simulink model "sampleModel1510_1_sub_sub"  (R2023a)
settings: Solver=VariableStepAuto  StartTime=0.0  StopTime=10.0  RelTol=1e-3
libraries: simulink x3, hdlsllib x1
settings Model: Creator=user1  LastModifiedBy=user1
settings OptimizationCC: BlockReduction=off  ConditionallyExecuteInputs=off

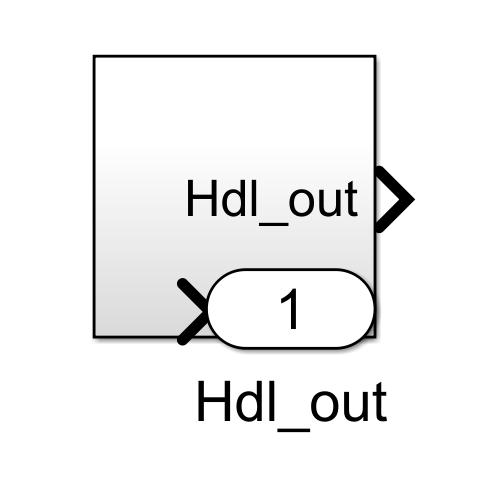
[thumbnail: Simulink's stored preview of the top-level diagram]
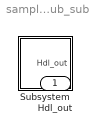
== system sampleModel1510_1_sub_sub ==
  Subsystem : Subsystem
  Hdl_out : Outport  OutDataTypeStr=uint8

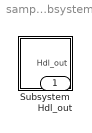
== system sampleModel1510_1_sub_sub/Subsystem ==
  Subsystem : Subsystem
  Hdl_out : Outport  OutDataTypeStr=uint8

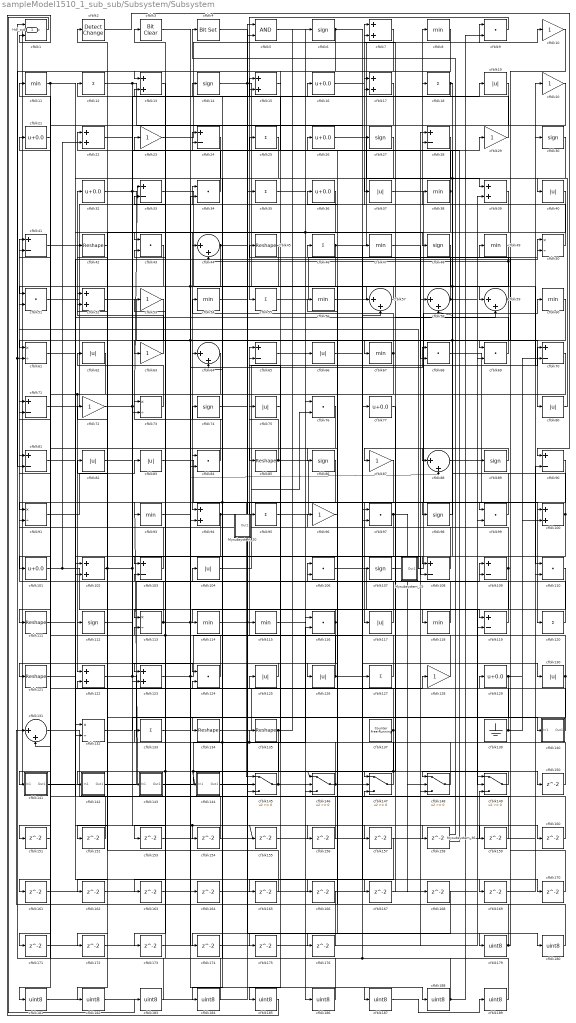
== system sampleModel1510_1_sub_sub/Subsystem/Subsystem ==
  Mysubsystem_20 : Subsystem  TreatAsAtomicUnit=on  RTWFcnName=Mysubsystem_20
      settings: RTWFcnNameOpts=User specified  RTWFileNameOpts=Use function name
  Mysubsystem_25 : Subsystem  TreatAsAtomicUnit=on  RTWFcnName=Mysubsystem_25
      settings: RTWFcnNameOpts=User specified  RTWFileNameOpts=Use function name
  Mysubsystem_36 : Subsystem  TreatAsAtomicUnit=on  RTWFcnName=Mysubsystem_36
      settings: RTWFcnNameOpts=User specified  RTWFileNameOpts=Use function name
  cfblk1 : RelationalOperator  Operator=<=  OutDataTypeStr=boolean  InputSameDT=off
  cfblk{10,20,23,29,53,63,72,87,96,128} (10 alike) : Gain  OutDataTypeStr=uint8
  cfblk{7,13,15,17,22,39,52,94,100,102,122..123} (12 alike) : Sum  OutDataTypeStr=uint8
  cfblk{16,21,26,32,36,77,101,129} (8 alike) : Bias  Bias=0.0  SaturateOnIntegerOverflow=off
  cfblk{24,28,33,41,65,70..71,81,90,103,108..109,119} (13 alike) : Sum  Inputs=+-  OutDataTypeStr=uint8
  cfblk{19,37,40,62,66,75,80,82..83,104,117,125..126,130} (14 alike) : Abs  OutDataTypeStr=uint8  SaturateOnIntegerOverflow=off
  cfblk{9,34,43,51,68..69,76,84,97,99,106,110,116,124} (14 alike) : DotProduct  OutDataTypeStr=uint8
  cfblk{6,14,27,30,48,74,86,89,98,107,112} (11 alike) : Signum
  cfblk{8,11,38,47,49,54,56,60,67,93,114..115,118} (13 alike) : MinMax  OutDataTypeStr=uint8
  cfblk{42,45,85,111,121,134..135} (7 alike) : Reshape
  cfblk{50,61,73,91,113,132} (6 alike) : Product  Inputs=*/  OutDataTypeStr=uint8  RndMeth=Zero  SaturateOnIntegerOverflow=on
  cfblk{12,18,25,35,46,55,95,120,127,133} (10 alike) : Sum  Inputs=+  OutDataTypeStr=uint8
  cfblk{44,57..59,64,88,131} (7 alike) : Sum  Inputs=|++  OutDataTypeStr=uint8
  cfblk137 : hdlsllib/Sources/Counter Free-Running  NumBits=16  tsamp=-1
  cfblk139 : Ground
  cfblk140 : Subsystem
      settings: LibrarySourceBlock=|
      | hdlsllib/Ports &
      | Subsystems/Subsystem
  cfblk141 : Subsystem
      settings: LibrarySourceBlock=|
      | hdlsllib/Ports &
      | Subsystems/Subsystem
  cfblk142 : Subsystem
      settings: LibrarySourceBlock=|
      | hdlsllib/Ports &
      | Subsystems/Subsystem
  cfblk143 : Subsystem
      settings: LibrarySourceBlock=|
      | hdlsllib/Ports &
      | Subsystems/Subsystem
  cfblk144 : Subsystem
      settings: LibrarySourceBlock=|
      | hdlsllib/Ports &
      | Subsystems/Subsystem
  cfblk{145..149} (5 alike) : Switch  OutDataTypeStr=uint8  SaturateOnIntegerOverflow=off  InputSameDT=off
  cfblk{150..176} (27 alike) : Delay  SampleTime=1
  cfblk{179..189} (11 alike) : DataTypeConversion  OutDataTypeStr=uint8  SaturateOnIntegerOverflow=off  RndMeth=Floor
  cfblk2 : simulink/Logic and Bit Operations/Detect Change  vinit=0  OutDataTypeStr=uint8
      settings: LibrarySourceBlock=|
      | hdlsllib/Logic and Bit
      | Operations/Detect
      | Change
  cfblk3 : simulink/Logic and Bit Operations/Bit Clear  iBit=0
      settings: LibrarySourceBlock=|
      | hdlsllib/Logic and Bit
      | Operations/Bit Clear
  cfblk4 : simulink/Logic and Bit Operations/Bit Set  iBit=0
      settings: LibrarySourceBlock=|
      | hdlsllib/Logic and Bit
      | Operations/Bit Set
  cfblk5 : Logic  AllPortsSameDT=off  OutDataTypeStr=boolean
  Hdl_out : Outport  OutDataTypeStr=uint8
  wires:
  Mysubsystem_36/2(Out2) -> cfblk23/1
  Mysubsystem_36/1(Out1) -> cfblk4/1
  Mysubsystem_25/1(Out1) -> cfblk51/2
  Mysubsystem_20/1(Out1) -> cfblk76/2
  cfblk189/1 -> cfblk133/1
  cfblk187/1 -> cfblk189/1
  cfblk188/1 -> cfblk97/1, cfblk74/1, cfblk9/2
  cfblk3/1 -> cfblk187/1
  cfblk186/1 -> cfblk3/1
  cfblk65/1 -> cfblk186/1
  cfblk185/1 -> cfblk1/2
  cfblk157/1 -> cfblk185/1
  cfblk184/1 -> cfblk1/1
  cfblk168/1 -> cfblk184/1
  cfblk183/1 -> cfblk21/1
  cfblk1/1 -> cfblk183/1
  cfblk182/1 -> cfblk5/2
  cfblk42/1 -> cfblk182/1
  cfblk181/1 -> cfblk5/1
  cfblk87/1 -> cfblk181/1
  cfblk180/1 -> cfblk36/1
  cfblk5/1 -> cfblk180/1
  cfblk179/1 -> cfblk113/2, cfblk129/1
  cfblk176/1 -> cfblk64/2
  cfblk175/1 -> cfblk58/1
  cfblk75/1 -> cfblk175/1
  cfblk174/1 -> cfblk148/3
  cfblk173/1 -> cfblk57/2
  cfblk172/1 -> cfblk39/2
  cfblk70/1 -> cfblk172/1
  cfblk171/1 -> cfblk34/2
  cfblk170/1 -> cfblk109/2
  cfblk169/1 -> cfblk110/2
  cfblk167/1 -> cfblk147/3
  cfblk166/1 -> cfblk131/1
  cfblk61/1 -> cfblk166/1
  cfblk165/1 -> cfblk122/2
  cfblk164/1 -> cfblk99/2
  cfblk93/1 -> cfblk164/1
  cfblk163/1 -> cfblk69/2
  cfblk162/1 -> cfblk149/1
  cfblk36/1 -> cfblk162/1
  cfblk161/1 -> cfblk28/1
  cfblk43/1 -> cfblk161/1
  cfblk160/1 -> cfblk7/2
  cfblk115/1 -> cfblk160/1
  cfblk159/1 -> cfblk71/2
  cfblk158/1 -> cfblk149/3
  cfblk156/1 -> cfblk132/1
  cfblk112/1 -> cfblk156/1
  cfblk155/1 -> cfblk97/2
  cfblk154/1 -> cfblk41/2
  cfblk153/1 -> cfblk90/2
  cfblk152/1 -> cfblk102/1
  cfblk151/1 -> cfblk91/2
  cfblk20/1 -> cfblk151/1
  cfblk150/1 -> cfblk65/2
  cfblk74/1 -> cfblk150/1
  cfblk137/1 -> cfblk73/1, cfblk146/3
  cfblk19/1 -> cfblk147/2
  cfblk64/1 -> cfblk131/2
  cfblk48/1 -> cfblk101/1
  cfblk97/1 -> cfblk102/2, cfblk148/2
  cfblk108/1 -> cfblk42/1
  cfblk148/1 -> cfblk135/1, cfblk82/1
  cfblk118/1 -> cfblk52/1
  cfblk119/1 -> cfblk13/2
  cfblk4/1 -> cfblk179/1
  cfblk28/1 -> cfblk37/1
  cfblk69/1 -> cfblk27/1
  cfblk60/1 -> cfblk113/1, cfblk84/2, cfblk108/1
  cfblk22/1 -> cfblk19/1
  cfblk88/1 -> cfblk89/1
  cfblk121/1 -> cfblk59/2
  cfblk2/1 -> cfblk90/1
  cfblk96/1 -> cfblk56/1
  cfblk7/1 -> cfblk85/1
  cfblk82/1 -> cfblk34/1
  cfblk47/1 -> cfblk68/2
  cfblk130/1 -> cfblk106/2, cfblk145/3
  cfblk49/1 -> cfblk58/2, cfblk176/1
  cfblk114/1 -> cfblk18/1, cfblk158/1
  cfblk29/1 -> cfblk2/1
  cfblk111/1 -> cfblk50/1
  cfblk126/1 -> cfblk53/1, cfblk11/1, cfblk169/1
  cfblk11/1 -> cfblk111/1, cfblk44/1
  cfblk40/1 -> cfblk145/2
  cfblk124/1 -> cfblk33/2
  cfblk30/1 -> cfblk84/1, cfblk88/1
  cfblk134/1 -> cfblk57/1
  cfblk135/1 -> cfblk152/1, cfblk153/1, cfblk6/1
  cfblk120/1 -> cfblk104/1
  cfblk103/1 -> cfblk81/1
  cfblk33/1 -> cfblk76/1
  cfblk66/1 -> cfblk130/1
  cfblk41/1 -> cfblk48/1
  cfblk67/1 -> cfblk54/1, cfblk163/1
  cfblk98/1 -> cfblk28/2
  cfblk76/1 -> cfblk141/1(In1)
  cfblk52/1 -> cfblk80/1
  cfblk34/1 -> cfblk12/1
  cfblk55/1 -> cfblk20/1
  cfblk8/1 -> cfblk61/2, cfblk81/2
  cfblk59/1 -> cfblk45/1, cfblk44/2, cfblk86/1
  cfblk100/1 -> cfblk24/1, cfblk123/1
  cfblk84/1 -> cfblk43/2
  cfblk57/1 -> cfblk51/1
  cfblk123/1 -> cfblk47/1, cfblk88/2
  cfblk26/1 -> cfblk39/1
  cfblk143/1(Out1) -> cfblk116/2, cfblk35/1, cfblk146/1
  cfblk109/1 -> cfblk14/1, cfblk165/1
  cfblk132/1 -> cfblk140/1(In1)
  cfblk80/1 -> cfblk40/1
  cfblk113/1 -> cfblk68/1, cfblk167/1, cfblk52/2
  cfblk91/1 -> cfblk83/1
  cfblk53/1 -> cfblk61/1
  cfblk85/1 -> cfblk127/1, cfblk75/1
  cfblk38/1 -> cfblk64/1, cfblk15/1
  cfblk99/1 -> cfblk25/1
  cfblk102/1 -> cfblk29/1, cfblk119/1, cfblk72/1
  cfblk23/1 -> cfblk9/1
  cfblk12/1 -> cfblk77/1, cfblk108/2
  cfblk101/1 -> cfblk149/2, cfblk22/2
  cfblk32/1 -> cfblk66/1, cfblk124/1
  cfblk25/1 -> cfblk134/1
  cfblk149/1 -> cfblk148/1
  cfblk146/1 -> cfblk62/1, cfblk124/2, cfblk70/1
  cfblk144/1(Out1) -> cfblk17/2
  cfblk44/1 -> cfblk94/2, cfblk123/2, cfblk107/1
  cfblk17/1 -> cfblk43/1
  cfblk110/1 -> cfblk126/1
  cfblk10/1 -> cfblk69/1
  cfblk145/1 -> cfblk103/2, cfblk159/1, Hdl_out/1
  cfblk21/1 -> cfblk91/1
  cfblk141/1(Out1) -> cfblk128/1
  cfblk133/1 -> cfblk188/1
  cfblk128/1 -> cfblk115/1
  cfblk94/1 -> cfblk112/1, cfblk157/1
  cfblk13/1 -> cfblk103/1
  cfblk45/1 -> cfblk94/1
  cfblk83/1 -> cfblk95/1
  cfblk62/1 -> cfblk122/1, cfblk171/1
  cfblk27/1 -> cfblk132/2
  cfblk56/1 -> cfblk59/1
  cfblk73/1 -> cfblk22/1
  cfblk116/1 -> cfblk114/1, cfblk26/1, cfblk173/1
  cfblk54/1 -> cfblk98/1
  cfblk16/1 -> cfblk17/1
  cfblk90/1 -> cfblk117/1
  cfblk51/1 -> cfblk38/1
  cfblk81/1 -> cfblk154/1, cfblk155/1
  cfblk6/1 -> cfblk13/1, cfblk119/2
  cfblk104/1 -> cfblk30/1
  cfblk39/1 -> cfblk93/1, cfblk146/2
  cfblk50/1 -> cfblk8/1
  cfblk122/1 -> cfblk109/1, cfblk24/2
  cfblk140/1(Out1) -> cfblk71/1
  cfblk129/1 -> cfblk142/1(In1), cfblk70/2
  cfblk14/1 -> cfblk110/1, cfblk170/1
  cfblk24/1 -> cfblk63/1
  cfblk71/1 -> cfblk7/1
  cfblk72/1 -> cfblk33/1, cfblk16/1
  cfblk106/1 -> cfblk118/1
  cfblk147/1 -> cfblk96/1, cfblk144/1(In1)
  cfblk117/1 -> cfblk41/1
  cfblk77/1 -> cfblk147/1
  cfblk107/1 -> cfblk60/1, cfblk168/1
  cfblk37/1 -> cfblk100/1
  cfblk127/1 -> cfblk65/1
  cfblk86/1 -> cfblk143/1(In1), cfblk174/1
  cfblk9/1 -> cfblk55/1
  cfblk68/1 -> cfblk120/1
  cfblk35/1 -> cfblk116/1
  cfblk142/1(Out1) -> cfblk106/1
  cfblk18/1 -> cfblk67/1, cfblk15/2
  cfblk46/1 -> cfblk10/1, cfblk73/2
  cfblk125/1 -> cfblk121/1
  cfblk58/1 -> cfblk46/1, cfblk50/2
  cfblk131/1 -> cfblk49/1
  cfblk63/1 -> cfblk32/1
  cfblk89/1 -> cfblk87/1
  cfblk15/1 -> cfblk145/1
  cfblk95/1 -> cfblk99/1
  cfblk139/1 -> cfblk125/1, cfblk100/2

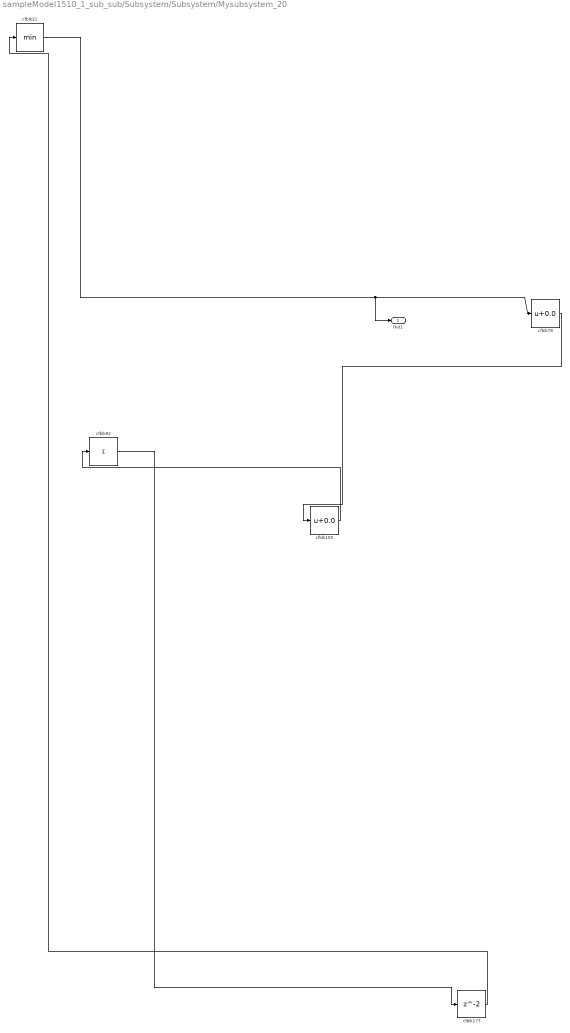
== system sampleModel1510_1_sub_sub/Subsystem/Subsystem/Mysubsystem_20 ==
  cfblk105 : Bias  Bias=0.0  SaturateOnIntegerOverflow=off
  cfblk177 : Delay  SampleTime=1
  cfblk31 : MinMax
  cfblk78 : Bias  Bias=0.0  SaturateOnIntegerOverflow=off
  cfblk92 : Sum  Inputs=+
  Out1 : Outport
  wires:
  cfblk105/1 -> cfblk92/1
  cfblk78/1 -> cfblk105/1
  cfblk31/1 -> Out1/1, cfblk78/1
  cfblk92/1 -> cfblk177/1
  cfblk177/1 -> cfblk31/1

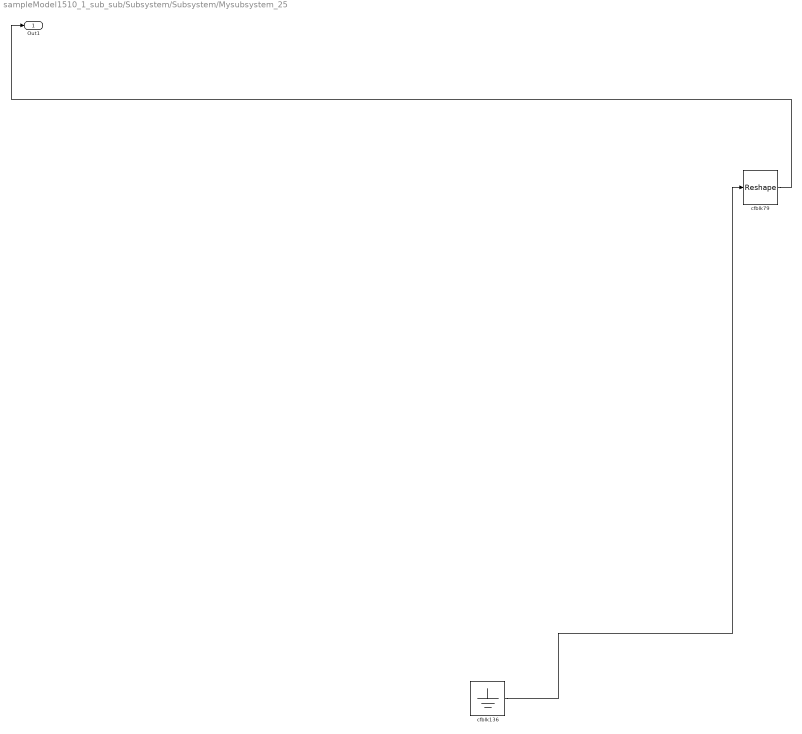
== system sampleModel1510_1_sub_sub/Subsystem/Subsystem/Mysubsystem_25 ==
  cfblk136 : Ground
  cfblk79 : Reshape
  Out1 : Outport
  wires:
  cfblk136/1 -> cfblk79/1
  cfblk79/1 -> Out1/1

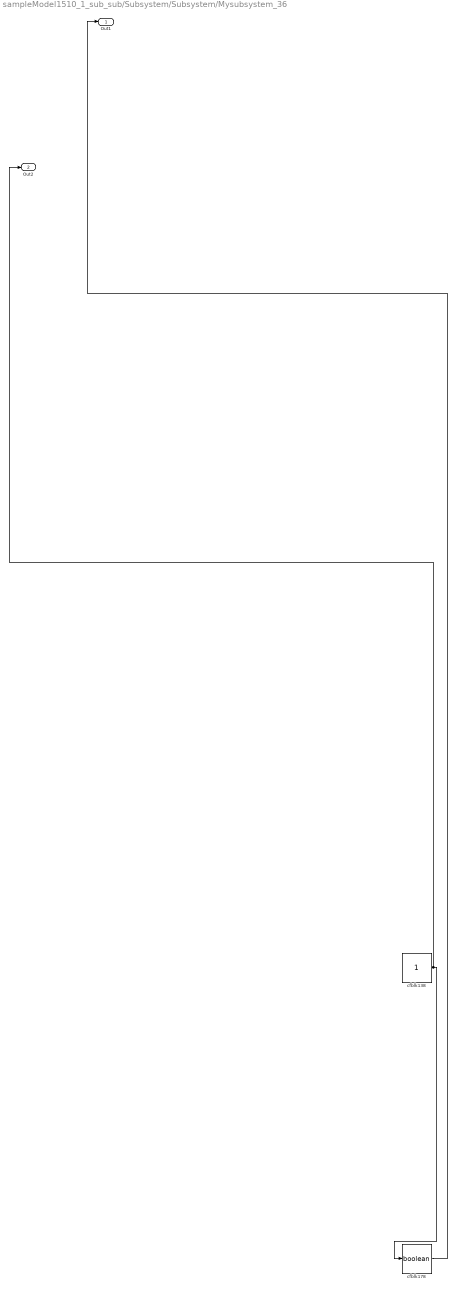
== system sampleModel1510_1_sub_sub/Subsystem/Subsystem/Mysubsystem_36 ==
  cfblk138 : Constant  SampleTime=-1
  cfblk178 : DataTypeConversion  OutDataTypeStr=boolean  SaturateOnIntegerOverflow=off  RndMeth=Floor
  Out1 : Outport
  Out2 : Outport  Port=2
  wires:
  cfblk138/1 -> Out2/1, cfblk178/1
  cfblk178/1 -> Out1/1

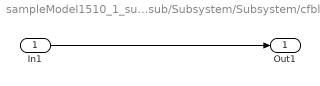
== system sampleModel1510_1_sub_sub/Subsystem/Subsystem/cfblk140 ==
  In1 : Inport
  Out1 : Outport
  wires:
  In1/1 -> Out1/1

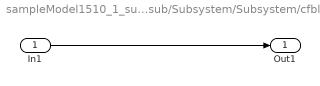
== system sampleModel1510_1_sub_sub/Subsystem/Subsystem/cfblk141 ==
  In1 : Inport
  Out1 : Outport
  wires:
  In1/1 -> Out1/1

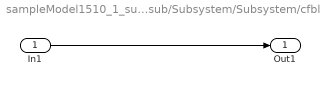
== system sampleModel1510_1_sub_sub/Subsystem/Subsystem/cfblk142 ==
  In1 : Inport
  Out1 : Outport
  wires:
  In1/1 -> Out1/1

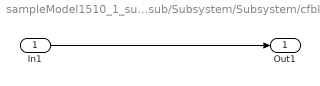
== system sampleModel1510_1_sub_sub/Subsystem/Subsystem/cfblk143 ==
  In1 : Inport
  Out1 : Outport
  wires:
  In1/1 -> Out1/1

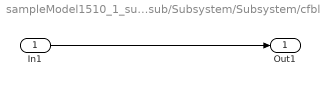
== system sampleModel1510_1_sub_sub/Subsystem/Subsystem/cfblk144 ==
  In1 : Inport
  Out1 : Outport
  wires:
  In1/1 -> Out1/1
